simulink model "xacc"  (R2020a)
settings: Solver=VariableStepAuto  StartTime=0.0  StopTime=10.0  RelTol=1e-3
undefined symbols (not defined in the file): Ax, m
settings Model: Creator=Muni Kumar  LastModifiedBy=Muni Kumar

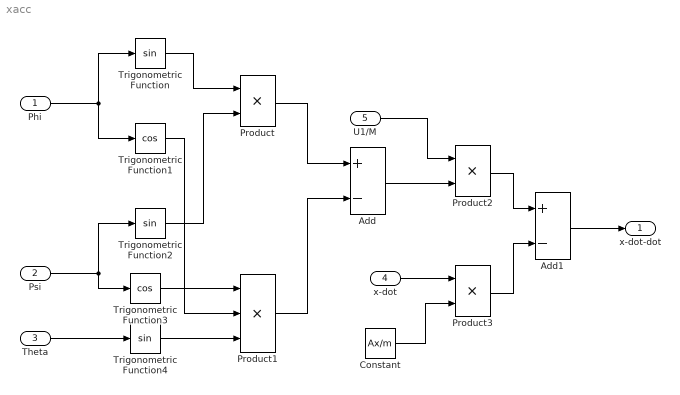
== system xacc ==
  Phi : Inport
  Psi : Inport  Port=2
  Theta : Inport  Port=3
  x-dot : Inport  Port=4
  U1/M : Inport  Port=5
  Add : Sum  Inputs=+-
  Add1 : Sum  Inputs=+-
  Constant : Constant  Value=Ax/m
  Product : Product
  Product1 : Product  Inputs=3
  Product2 : Product
  Product3 : Product
  Trigonometric Function : Trigonometry
  Trigonometric Function1 : Trigonometry  Operator=cos
  Trigonometric Function2 : Trigonometry
  Trigonometric Function3 : Trigonometry  Operator=cos
  Trigonometric Function4 : Trigonometry
  x-dot-dot : Outport
  wires:
  Trigonometric Function/1 -> Product/1
  Phi/1 -> Trigonometric Function1/1, Trigonometric Function/1
  Psi/1 -> Trigonometric Function3/1, Trigonometric Function2/1
  Trigonometric Function4/1 -> Product1/3
  Theta/1 -> Trigonometric Function4/1
  Trigonometric Function2/1 -> Product/2
  Trigonometric Function1/1 -> Product1/2
  Trigonometric Function3/1 -> Product1/1
  Product/1 -> Add/1
  Product1/1 -> Add/2
  x-dot/1 -> Product3/1
  Constant/1 -> Product3/2
  U1/M/1 -> Product2/1
  Add/1 -> Product2/2
  Product3/1 -> Add1/2
  Product2/1 -> Add1/1
  Add1/1 -> x-dot-dot/1
